simulink model "mass_spring_damper_model_ODE"  (Simulink 6.6)
settings: Solver=ode45  StartTime=0.0  StopTime=10.0  RelTol=1e-3
settings Model: Creator=lum  LastModifiedBy=lum

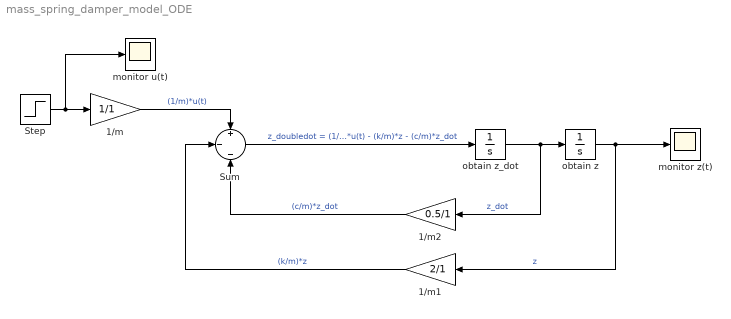
== system mass_spring_damper_model_ODE ==
  1/m : Gain  Gain=1/1
  1/m1 : Gain  Orientation=left  Gain=2/1
  1/m2 : Gain  Orientation=left  Gain=0.5/1
  Step : Step  SampleTime=0
  Sum : Sum  Inputs=+|-|-
  monitor u(t) : Scope
  monitor z(t) : Scope
      settings: TimeRange=10
  obtain z : Integrator
  obtain z_dot : Integrator
  wires:
  obtain z_dot/1 -> obtain z/1, 1/m2/1  "z_dot"
  obtain z/1 -> 1/m1/1, monitor z(t)/1  "z"
  Step/1 -> 1/m/1, monitor u(t)/1
  1/m2/1 -> Sum/3  "(c/m)*z_dot"
  1/m1/1 -> Sum/2  "(k/m)*z"
  1/m/1 -> Sum/1  "(1/m)*u(t)"
  Sum/1 -> obtain z_dot/1  "z_doubledot = (1/m)*u(t) - (k/m)*z - (c/m)*z_dot"
